simulink model "model_lab4"  (R2016b)
settings: Solver=ode23s  StartTime=0.0  StopTime=2  RelTol=1e-3
values from neighbouring files (symbols this model uses):
  A = [a12*X(3), a11, a12*X(1) ... (first row only)    [lab4.m]
  B = [a13 0 ... (first row only)    [lab4.m]
  i_n = 50    [lab4.m]
  J = 0.1    [lab4.m]
  x0 = [0,0,0]    [lab4.m]
undefined symbols (not defined in the file or in its folder): Ce, Cm, F_n, fi_n, La, Mb, om_n, R0, Ra, Rb, W
settings Model: Creator=khanh  LastModifiedBy=khanh

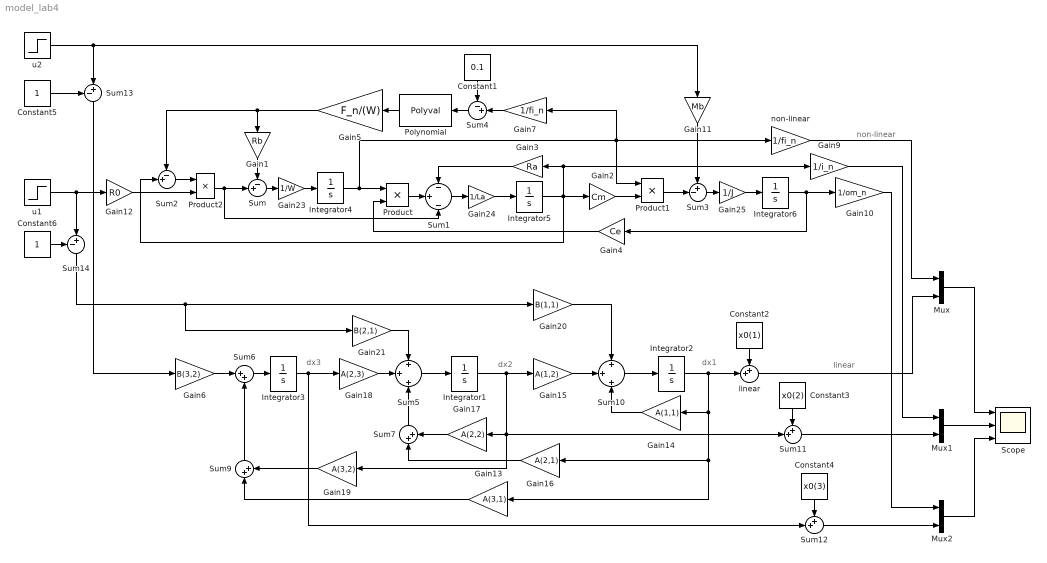
== system model_lab4 ==
  note: non-linear
  note: linear
  note: dx3
  note: dx2
  note: dx1
  Constant1 : Constant  Value=0.1
  Constant2 : Constant  Value=x0(1)
  Constant3 : Constant  Value=x0(2)
  Constant4 : Constant  Value=x0(3)
  Constant5 : Constant
  Constant6 : Constant
  Gain1 : Gain  Gain=Rb
  Gain10 : Gain  Gain=1/om_n
  Gain11 : Gain  Gain=Mb
  Gain12 : Gain  Gain=R0
  Gain13 : Gain  Gain=A(3,1)
  Gain14 : Gain  Gain=A(1,1)
  Gain15 : Gain  Gain=A(1,2)
  Gain16 : Gain  Gain=A(2,1)
  Gain17 : Gain  Gain=A(2,2)
  Gain18 : Gain  Gain=A(2,3)
  Gain19 : Gain  Gain=A(3,2)
  Gain2 : Gain  Gain=Cm
  Gain20 : Gain  Gain=B(1,1)
  Gain21 : Gain  Gain=B(2,1)
  Gain23 : Gain  Gain=1/W
  Gain24 : Gain  Gain=1/La
  Gain25 : Gain  Gain=1/J
  Gain3 : Gain  Gain=Ra
  Gain4 : Gain  Gain=Ce
  Gain5 : Gain  Gain=F_n/(W)
  Gain6 : Gain  Gain=B(3,2)
  Gain7 : Gain  Gain=1/fi_n
  Gain9 : Gain  Gain=1/i_n
  Integrator1 : Integrator  InitialCondition=x0(2)*0
  Integrator2 : Integrator  InitialCondition=x0(1)*0
  Integrator3 : Integrator  InitialCondition=x0(3)*0
  Integrator4 : Integrator  InitialCondition=x0(1)*fi_n*1
  Integrator5 : Integrator  InitialCondition=x0(2)*i_n*1
  Integrator6 : Integrator  InitialCondition=x0(3)*om_n*1
  Mux : Mux  Inputs=2
  Mux1 : Mux  Inputs=2
  Mux2 : Mux  Inputs=2
  Polynomial : Polyval  Coefs=[0.5176, 0, 0.9659, 0]
  Product : Product
  Product1 : Product
  Product2 : Product
  Scope : Scope  NumInputPorts=3
  Sum{,2,4,13..14} (5 alike) : Sum  Inputs=-+|
  Sum1 : Sum  Inputs=-|+|-
  Sum10 : Sum  Inputs=+|+|+
  Sum11 : Sum  Inputs=++|
  Sum12 : Sum  Inputs=++|
  Sum3 : Sum  Inputs=+-|
  Sum5 : Sum  Inputs=+|+|+
  Sum6 : Sum  Inputs=|++
  Sum7 : Sum  Inputs=|++
  Sum9 : Sum  Inputs=|++
  linear : Sum  Inputs=++|
  non-linear : Gain  Gain=1/fi_n
  u1 : Step  Time=0  After=1.1  SampleTime=0
  u2 : Step  Time=0  SampleTime=0
  wires:
  Product2/1 -> Sum1/3, Sum/2
  Gain1/1 -> Sum/1
  Product/1 -> Sum1/2
  Sum1/1 -> Gain24/1
  Gain3/1 -> Sum1/1
  Integrator5/1 -> Gain2/1, Gain9/1, Gain3/1, Sum2/2
  Gain4/1 -> Product/2
  Integrator4/1 -> Product/1, Product1/1, Gain7/1, non-linear/1
  Gain2/1 -> Product1/2
  Product1/1 -> Sum3/2
  Constant1/1 -> Sum4/1
  Gain5/1 -> Sum2/1, Gain1/1
  Sum4/1 -> Polynomial/1
  Polynomial/1 -> Gain5/1
  Integrator6/1 -> Gain4/1, Gain10/1
  Gain7/1 -> Sum4/2
  Sum2/1 -> Product2/1
  Gain11/1 -> Sum3/1
  Gain12/1 -> Product2/2
  Sum6/1 -> Integrator3/1
  Sum5/1 -> Integrator1/1
  Sum10/1 -> Integrator2/1
  Integrator2/1 -> linear/2, Gain13/1, Gain16/1, Gain14/1
  Gain14/1 -> Sum10/3
  Gain18/1 -> Sum5/2
  Gain19/1 -> Sum9/2
  Gain13/1 -> Sum9/1
  Gain15/1 -> Sum10/2
  Sum14/1 -> Gain21/1, Gain20/1
  Gain20/1 -> Sum10/1
  Sum9/1 -> Sum6/2
  Gain6/1 -> Sum6/1
  Gain21/1 -> Sum5/1
  Sum13/1 -> Gain6/1
  u2/1 -> Gain11/1, Sum13/2
  Sum7/1 -> Sum5/3
  Gain17/1 -> Sum7/2
  Gain16/1 -> Sum7/1
  Constant2/1 -> linear/1
  Integrator1/1 -> Gain15/1, Gain17/1, Sum11/2, Gain19/1
  Constant3/1 -> Sum11/1
  Integrator3/1 -> Gain18/1, Sum12/2
  Constant4/1 -> Sum12/1
  Sum/1 -> Gain23/1
  Gain23/1 -> Integrator4/1
  Gain24/1 -> Integrator5/1
  Gain25/1 -> Integrator6/1
  Sum3/1 -> Gain25/1
  non-linear/1 -> Mux/1
  linear/1 -> Mux/2
  Gain9/1 -> Mux1/1
  Sum11/1 -> Mux1/2
  Sum12/1 -> Mux2/2
  Gain10/1 -> Mux2/1
  Mux/1 -> Scope/1
  Mux1/1 -> Scope/2
  Mux2/1 -> Scope/3
  Constant5/1 -> Sum13/1
  u1/1 -> Gain12/1, Sum14/2
  Constant6/1 -> Sum14/1
